simulink model "MDCC"  (R2021b)
settings: Solver=FixedStepDiscrete  StartTime=0.0  StopTime=10.0  FixedStep=0.0001  RelTol=1e-3
model workspace (MATLAB code in the model file):
  | cmdLim = Simulink.Parameter;
  | cmdLim.Value = 15;
  | cmdLim.Description = 'Limit for controlling the maximum surface command angle.';
  | cmdLim.Min = 0;
  | cmdLim.Max = 90;
  | cmdLim.DocUnits = 'deg';
  | 
  | dispGain = Simulink.Parameter;
  | dispGain.Value = 0.75;
  | dispGain.Description = 'Gain applied to the displacement error.';
  | dispGain.Min = 0;
  | dispGain.Max = [];
  | dispGain.DocUnits = 'deg/sec/deg';
  | 
  | dispLim = Simulink.Parameter;
  | dispLim.Value = 30;
  | dispLim.Description = 'Limit for controlling the maximum commanded angle.';
  | dispLim.Min = 0;
  | dispLim.Max = 180;
  | dispLim.DocUnits = 'deg';
  | 
  | intGain = Simulink.Parameter;
  | intGain.Value = 0.5;
  | intGain.Description = 'Gain applied to the integral error.';
  | intGain.Min = 0;
  | intGain.Max = [];
  | intGain.DocUnits = 'deg/sec/deg/sec';
  | 
  | intLim = Simulink.Parameter;
  | intLim.Value = 5;
  | intLim.Description = 'Limit for controlling the maximum commanded angle.';
  | intLim.Min = 0;
  | intLim.Max = 90;
  | intLim.DocUnits = 'deg';
  | 
  | rateGain = Simulink.Parameter;
  | rateGain.Value = 2;
  | rateGain.Description = 'Gain applied to the rate error.';
  | rateGain.Min = 0;
  | rateGain.Max = [];
  | rateGain.DocUnits = 'deg/deg/sec';
  | 
  | rateLim = Simulink.Parameter;
  | rateLim.Value = 6;
  | rateLim.Description = 'Limit for controlling the maximum commanded angle.';
  | rateLim.Min = 0;
  | rateLim.Max = 180;
  | rateLim.DocUnits = 'deg/sec';
  | 
  | hdgGain = Simulink.Parameter;
  | hdgGain.Value = 0.015;
values from neighbouring files (symbols this model uses):
  KfDeadCompen_SetDeltaTime_us = myPackage.Parameter    [DeadCompen.m]
  Ts = 5E-6    (= 5e-06)    [iPMSM_data.m]
  VbDeadComp_SwtUseIsttrDes_flg = myPackage.Parameter    [DeadCompen.m]
  VfDeadCompen_ISttrDdeThdSwt_A = myPackage.Parameter    [DeadCompen.m]
  VfDeadCompen_ISttrIgbtThdSwt_A = myPackage.Parameter    [DeadCompen.m]
  VfDeadCompen_rDdeISttrHi_R = myPackage.Parameter    [DeadCompen.m]
  VfDeadCompen_rDdeISttrLo_R = myPackage.Parameter    [DeadCompen.m]
  VfDeadCompen_rIgbtISttrHi_R = myPackage.Parameter    [DeadCompen.m]
  VfDeadCompen_rIgbtISttrLo_R = myPackage.Parameter    [DeadCompen.m]
  VfDeadCompen_uDdeISttrHi_V = myPackage.Parameter    [DeadCompen.m]
  VfDeadCompen_uDdeISttrLo_V = myPackage.Parameter    [DeadCompen.m]
  VfDeadCompen_uIgbtISttrHi_V = myPackage.Parameter    [DeadCompen.m]
  VfDeadCompen_uIgbtISttrLo_V = myPackage.Parameter    [DeadCompen.m]
undefined symbols (not defined in the file or in its folder): CosTable12bit_Y, GLBCal_GLBCal_Kf_DCLinkOverVolErrThd_V, GLBCal_GLBCal_Kf_DCLinkUnderVolErrThd_V, GLBCal_GLBCal_Kf_EquiLd_NULL, GLBCal_GLBCal_Kf_EquiLq_NULL, GLBCal_GLBCal_Kf_MotorRatedSpeed_rpm, GLBCal_GLBCal_Kf_MotorSpeedHysteresis_Coef, GLBCal_Ke_MotorPolePairsNum_NULL, IoHwAbOpArg_PwmDutyCyclePhU_NULL, IoHwAbOpArg_PwmDutyCyclePhV_NULL, IoHwAbOpArg_PwmDutyCyclePhW_NULL, IoHwAbOpArg_PwmOutputEn, KbMDCC_DeadTimeCompEn_flg, KbMDCC_MCF_flgHarmInIsdqTab11ZR_flg, KbMDCC_MCF_flgHarmInIsdqTab13ZR_flg, KbMDCC_MCF_flgHarmInIsdqTab5ZR_flg, KbMDCC_MCF_flgHarmInIsdqTab7ZR_flg, KbMDCC_MCF_flgHarmInject_flg, KbMDCC_SetEAngleEn_flg, KbMDCC_UdUqFwOmit_flg, KfDeadCompen_CpPeriodTimesT_NULL, KfMDCC_ActiveDischargeIdCurVal_A, KfMDCC_ActiveDischargeIqCurVal_A, KfMDCC_DCLinkVolRate_coef, KfMDCC_DebugEAngleInit_rad, KfMDCC_DebugUalphaVolCmd_V, KfMDCC_DebugUbetaVolCmd_V, KfMDCC_DebugUdCmd_V, KfMDCC_DebugUqCmd_V, KfMDCC_DebugUsCmd_V, KfMDCC_DebugUsRate_V, KfMDCC_IMCResp_NULL, KfMDCC_IMCStab_NULL, KfMDCC_InvParkCpPeriodTimesT_NULL, KfMDCC_MCF_CircAge_NULL, KfMDCC_MCF_flgUse11Harm_flg, KfMDCC_MCF_flgUse13Harm_flg, KfMDCC_MCF_flgUse5Harm_flg, KfMDCC_MCF_flgUse7Harm_flg, KfMDCC_MCF_Harm1113FLParamSpeedThrd_rads, KfMDCC_MCF_Harm57FLParamSpeedThrd_rads, KfMDCC_MCF_HarmcofFltN_NULL, KfMDCC_MCF_HarmCpnAg_NULL, KfMDCC_MCF_HarmfLParaHigh_coef, KfMDCC_MCF_HarmfLParaLow_coef, KfMDCC_MCF_HarmIn1113ZRY_Trq_Nm, KfMDCC_MCF_HarmIn11_SpdLimHigh_rads, KfMDCC_MCF_HarmIn11_SpdLimLow_rads, KfMDCC_MCF_HarmIn11ZRY_Isd_A, KfMDCC_MCF_HarmIn11ZRY_Isq_A, KfMDCC_MCF_HarmIn13_SpdLimHigh_rads, KfMDCC_MCF_HarmIn13_SpdLimLow_rads, KfMDCC_MCF_HarmIn13ZRY_Isd_A, KfMDCC_MCF_HarmIn13ZRY_Isq_A, KfMDCC_MCF_HarmIn57ZRY_Trq_Nm, KfMDCC_MCF_HarmIn5_SpdLimHigh_rads, KfMDCC_MCF_HarmIn5_SpdLimLow_rads, KfMDCC_MCF_HarmIn5ZRY_Isd_A, KfMDCC_MCF_HarmIn5ZRY_Isq_A, KfMDCC_MCF_HarmIn7_SpdLimHigh_rads ... (+47)
libraries: simulink x40, PMSM_Library x3, mcbcontrolslib x1
(part 1 of 8)
settings Model: RequirementInfo={} %GIDa_fe9045fd_0412_4b6e_8206_617cc20e6fde  DataDictionary=MDCC_Merge.sldd  FPTRunName=Active  Creator=洲  LastModifiedBy=洲
settings SolverCC: AlgebraicLoopSolver=TrustRegion  AutoInsertRateTranBlk=on
settings DataIOCC: SaveOutput=off  SignalLogging=off  DSMLogging=off  SaveTime=off
settings OptimizationCC: DefaultParameterBehavior=Inlined  UseDivisionForNetSlopeComputation=on  GainParamInheritBuiltInType=on  UseFloatMulNetSlope=on  DefaultUnderspecifiedDataType=single  UseSpecifiedMinMax=on  StrengthReduction=on  PassReuseOutputArgsAs=Individual arguments  ZeroExternalMemoryAtStartup=off  ZeroInternalMemoryAtStartup=off  NoFixptDivByZeroProtection=on  EfficientFloat2IntCast=on  OptimizeBlockOrder=speed  OptimizationPriority=Speed  OptimizationCustomize=off  MultiThreadedLoops=on  EfficientTunableParamExpr=on
settings DebuggingCC: ParameterTunabilityLossMsg=error  SFUnexpectedBacktrackingDiag=warning  SFNoUnconditionalDefaultTransitionDiag=warning  SFExecutionAtInitializationDiag=none  ArithmeticOperatorsInVariantConditions=warning
settings HardwareCC: ProdBitPerPointer=32  ProdBitPerSizeT=32  ProdBitPerPtrDiffT=32  ProdLargestAtomicInteger=Long  ProdLargestAtomicFloat=Double  ProdEndianess=BigEndian  ProdWordSize=32  ProdLongLongMode=on  ProdHWDeviceType=Freescale->32-bit PowerPC
settings ModelReferenceCC: ModelReferenceNumInstancesAllowed=Single
settings SFSimCC: MATLABDynamicMemAlloc=off  CustomCodeUndefinedFunction=UseInterfaceOnly
settings RTWCC: Description=AUTOSAR  SystemTargetFile=autosar.tlc  GenCodeOnly=on  TemplateMakefile=ert_default_tmf  BuildConfiguration=Faster Runs
settings CodeAppCC: ForceParamTrailComments=on  IgnoreCustomStorageClasses=off  MaxIdLength=128  OperatorAnnotations=on  SimulinkDataObjDesc=on  SFDataObjDesc=on  InsertBlockDesc=on  ReqsInCode=on
settings STFCustomTargetCC: TargetLangStandard=C99 (ISO)  UtilityFuncGeneration=Shared location  MultiwordLength=256  ParMdlRefBuildCompliant=on  CompOptLevelCompliant=on  IncludeMdlTerminateFcn=off  CombineOutputUpdateFcns=on  SuppressErrorStatus=on  ERTCustomFileBanners=on  SupportNonFinite=off  SupportComplex=off  SupportContinuousTime=off  SupportNonInlinedSFcns=off  RemoveResetFunc=on  MATLABClassNameForMDSCustomization=Simulink.SoftwareTarget.ERTCustomization  AutosarCompliant=on  GRTInterface=off  UseToolchainInfoCompliant=on  LookupTableObjectStructAxisOrder=2,1,3,4,...  LUTObjectStructOrderEvenSpacing=Size,Table,Breakpoints  SystemTargetFile=autosar.tlc
settings ERTTargetCC: TargetLangStandard=C99 (ISO)  UtilityFuncGeneration=Shared location  ConcurrentExecutionCompliant=off  IncludeMdlTerminateFcn=off  SuppressErrorStatus=on  SupportNonFinite=off  SupportComplex=off  ModelStepFunctionPrototypeControlCompliant=off  CPPClassGenCompliant=off  AutosarCompliant=on  LookupTableObjectStructAxisOrder=2,1,3,4,...  LUTObjectStructOrderEvenSpacing=Size,Table,Breakpoints  GenerateASAP2=on  InlinedParameterPlacement=NonHierarchical  ERTCustomFileTemplate=example_file_process.tlc
settings ConfigComp: CovScope=ReferencedModels  CovSaveName=covdata_rollAP  CovMetricSettings=dcmtrwe  CovHTMLOptions=-sRT=1 -aTS=1 -bRG=1 -bTC=1 -hTR=1 -nFC=0 -scm=1 -bcm=1 -xEv=0  CovSaveCumulativeToWorkspaceVar=on  CovSaveSingleToWorkspaceVar=on  CovCumulativeVarName=covCumulativeData_rollAP  CovReportOnPause=off  CovExternalEMLEnable=off  CovSFcnEnable=off

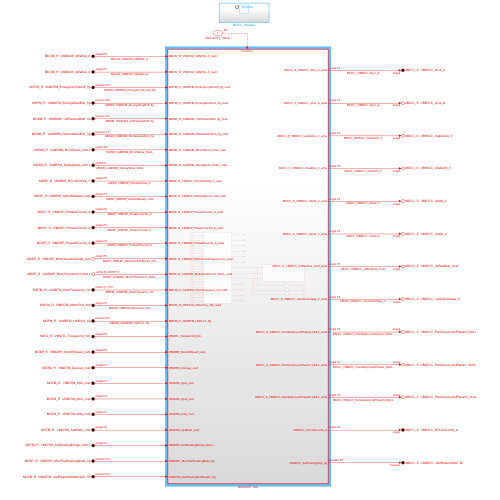
[thumbnail: Simulink's stored preview of the top-level diagram]
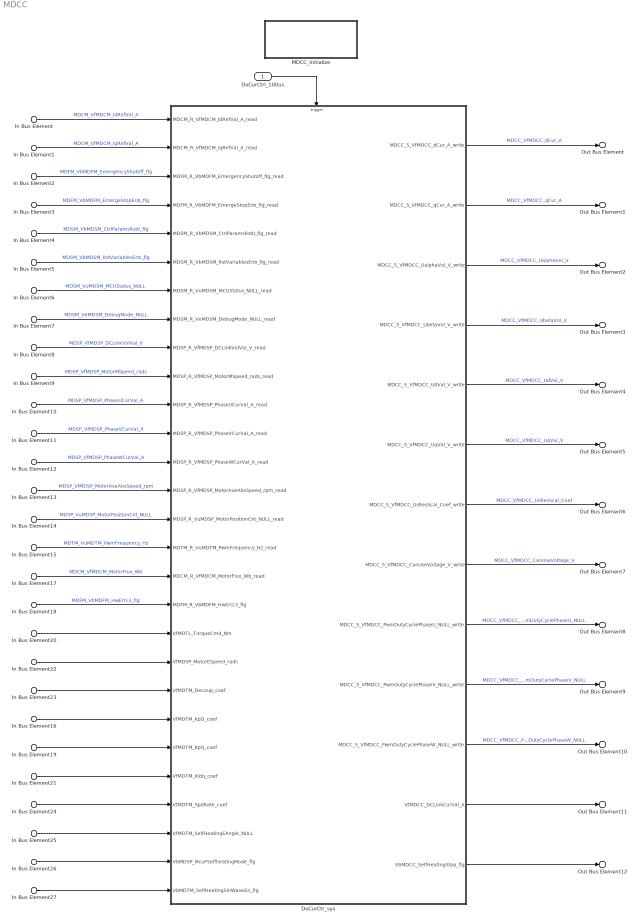
== system MDCC ==
  DoCurCtrl_100us : Inport  SampleTime=0.0001  OutputFunctionCall=on
  In Bus Element : Inport  Port=2  PortName=MDCM_R  Element=VfMDCM_IdRefVal_A
  In Bus Element1 : Inport  Port=2  PortName=MDCM_R  Element=VfMDCM_IqRefVal_A
  In Bus Element17 : Inport  Port=2  PortName=MDCM_R  Element=VfMDCM_MotorFlux_Wb
  In Bus Element2 : Inport  Port=3  PortName=MDFM_R  Element=VbMDFM_EmergencyShutoff_flg
  In Bus Element3 : Inport  Port=3  PortName=MDFM_R  Element=VbMDFM_EmergeStopEnb_flg
  In Bus Element18 : Inport  Port=3  PortName=MDFM_R  Element=VbMDFM_HwErrL3_flg
  In Bus Element4 : Inport  Port=4  PortName=MDSM_R  Element=VbMDSM_CtrlParamsRst0_flg
  In Bus Element5 : Inport  Port=4  PortName=MDSM_R  Element=VbMDSM_RstVariablesEnb_flg
  In Bus Element7 : Inport  Port=4  PortName=MDSM_R  Element=VeMDSM_DebugMode_NULL
  In Bus Element6 : Inport  Port=4  PortName=MDSM_R  Element=VuMDSM_MCUStatus_NULL
  In Bus Element26 : Inport  Port=5  PortName=MDSP_R  Element=VbMDSP_McuFSelfheatingMode_flg
  In Bus Element8 : Inport  Port=5  PortName=MDSP_R  Element=VfMDSP_DCLinkVolVal_V
  In Bus Element13 : Inport  Port=5  PortName=MDSP_R  Element=VfMDSP_MotorAveAbsSpeed_rpm
  In Bus Element22 : Inport  Port=5  PortName=MDSP_R  Element=VfMDSP_MotorESpeed_rads
  In Bus Element9 : Inport  Port=5  PortName=MDSP_R  Element=VfMDSP_MotorMSpeed_rads
  In Bus Element10 : Inport  Port=5  PortName=MDSP_R  Element=VfMDSP_PhaseUCurVal_A
  In Bus Element11 : Inport  Port=5  PortName=MDSP_R  Element=VfMDSP_PhaseVCurVal_A
  In Bus Element12 : Inport  Port=5  PortName=MDSP_R  Element=VfMDSP_PhaseWCurVal_A
  In Bus Element14 : Inport  Port=5  PortName=MDSP_R  Element=VuMDSP_MotorPositionCnt_NULL
  In Bus Element27 : Inport  Port=6  PortName=MDTM_R  Element=VbMDTM_SelfHeatingSinWaveEn_flg
  In Bus Element25 : Inport  Port=6  PortName=MDTM_R  Element=VfMDTM_SelfHeatingEAngle_NULL
  In Bus Element16 : Inport  Port=6  PortName=MDTM_R  Element=VfMDTM_KpD_coef
  In Bus Element19 : Inport  Port=6  PortName=MDTM_R  Element=VfMDTM_KpQ_coef
  In Bus Element21 : Inport  Port=6  PortName=MDTM_R  Element=VfMDTM_Kidq_coef
  In Bus Element23 : Inport  Port=6  PortName=MDTM_R  Element=VfMDTM_Decoup_coef
  In Bus Element24 : Inport  Port=6  PortName=MDTM_R  Element=VfMDTM_SpdRate_coef
  In Bus Element15 : Inport  Port=6  PortName=MDTM_R  Element=VuMDTM_PwmFrequency_Hz
  In Bus Element20 : Inport  Port=7  PortName=MDTL_R  Element=VfMDTL_TorqueCmd_Nm
  DoCurCtr_sys : Subsystem  Description=""
      settings: AttributesFormatString=%<Description>
  MDCC_Initialize : Subsystem  TreatAsAtomicUnit=on
  Out Bus Element12 : Outport  PortName=MDCC_S  Element=VbMDCC_SelfHeatingStop_flg
  Out Bus Element11 : Outport  PortName=MDCC_S  Element=VfMDCC_DCLinkCurVal_A
  Out Bus Element9 : Outport  PortName=MDCC_S  Element=VfMDCC_PwmDutyCyclePhaseV_NULL
  Out Bus Element7 : Outport  PortName=MDCC_S  Element=VfMDCC_CanUseVoltage_V
  Out Bus Element : Outport  PortName=MDCC_S  Element=VfMDCC_dCur_A
  Out Bus Element8 : Outport  PortName=MDCC_S  Element=VfMDCC_PwmDutyCyclePhaseU_NULL
  Out Bus Element10 : Outport  PortName=MDCC_S  Element=VfMDCC_PwmDutyCyclePhaseW_NULL
  Out Bus Element1 : Outport  PortName=MDCC_S  Element=VfMDCC_qCur_A
  Out Bus Element2 : Outport  PortName=MDCC_S  Element=VfMDCC_UalphaVol_V
  Out Bus Element3 : Outport  PortName=MDCC_S  Element=VfMDCC_UbetaVol_V
  Out Bus Element4 : Outport  PortName=MDCC_S  Element=VfMDCC_UdVal_V
  Out Bus Element5 : Outport  PortName=MDCC_S  Element=VfMDCC_UqVal_V
  Out Bus Element6 : Outport  PortName=MDCC_S  Element=VfMDCC_UsResScal_Coef
  wires:
  DoCurCtr_sys/10(MDCC_S_VfMDCC_PwmDutyCyclePhaseV_NULL_write) -> Out Bus Element9/1  "MDCC_VfMDCC_PwmDutyCyclePhaseV_NULL"
  DoCurCtr_sys/9(MDCC_S_VfMDCC_PwmDutyCyclePhaseU_NULL_write) -> Out Bus Element8/1  "MDCC_VfMDCC_PwmDutyCyclePhaseU_NULL"
  DoCurCtr_sys/3(MDCC_S_VfMDCC_UalphaVol_V_write) -> Out Bus Element2/1  "MDCC_VfMDCC_UalphaVol_V"
  In Bus Element14/1 -> DoCurCtr_sys/15(MDSP_R_VuMDSP_MotorPositionCnt_NULL_read)  "MDSP_VuMDSP_MotorPositionCnt_NULL"
  In Bus Element18/1 -> DoCurCtr_sys/18(MDFM_R_VbMDFM_HwErrL3_flg)  "MDFM_VbMDFM_HwErrL3_flg"
  DoCurCtr_sys/11(MDCC_S_VfMDCC_PwmDutyCyclePhaseW_NULL_write) -> Out Bus Element10/1  "MDCC_VfMDCC_PwmDutyCyclePhaseW_NULL"
  In Bus Element/1 -> DoCurCtr_sys/1(MDCM_R_VfMDCM_IdRefVal_A_read)  "MDCM_VfMDCM_IdRefVal_A"
  In Bus Element7/1 -> DoCurCtr_sys/8(MDSM_R_VeMDSM_DebugMode_NULL_read)  "MDSM_VeMDSM_DebugMode_NULL"
  In Bus Element11/1 -> DoCurCtr_sys/12(MDSP_R_VfMDSP_PhaseVCurVal_A_read)  "MDSP_VfMDSP_PhaseVCurVal_A"
  In Bus Element13/1 -> DoCurCtr_sys/14(MDSP_R_VfMDSP_MotorAveAbsSpeed_rpm_read)  "MDSP_VfMDSP_MotorAveAbsSpeed_rpm"
  DoCurCtr_sys/6(MDCC_S_VfMDCC_UqVal_V_write) -> Out Bus Element5/1  "MDCC_VfMDCC_UqVal_V"
  DoCurCtr_sys/4(MDCC_S_VfMDCC_UbetaVol_V_write) -> Out Bus Element3/1  "MDCC_VfMDCC_UbetaVol_V"
  In Bus Element1/1 -> DoCurCtr_sys/2(MDCM_R_VfMDCM_IqRefVal_A_read)  "MDCM_VfMDCM_IqRefVal_A"
  In Bus Element8/1 -> DoCurCtr_sys/9(MDSP_R_VfMDSP_DCLinkVolVal_V_read)  "MDSP_VfMDSP_DCLinkVolVal_V"
  DoCurCtr_sys/7(MDCC_S_VfMDCC_UsResScal_Coef_write) -> Out Bus Element6/1  "MDCC_VfMDCC_UsResScal_Coef"
  In Bus Element10/1 -> DoCurCtr_sys/11(MDSP_R_VfMDSP_PhaseUCurVal_A_read)  "MDSP_VfMDSP_PhaseUCurVal_A"
  DoCurCtr_sys/1(MDCC_S_VfMDCC_dCur_A_write) -> Out Bus Element/1  "MDCC_VfMDCC_dCur_A"
  In Bus Element9/1 -> DoCurCtr_sys/10(MDSP_R_VfMDSP_MotorMSpeed_rads_read)  "MDSP_VfMDSP_MotorMSpeed_rads"
  DoCurCtr_sys/5(MDCC_S_VfMDCC_UdVal_V_write) -> Out Bus Element4/1  "MDCC_VfMDCC_UdVal_V"
  In Bus Element12/1 -> DoCurCtr_sys/13(MDSP_R_VfMDSP_PhaseWCurVal_A_read)  "MDSP_VfMDSP_PhaseWCurVal_A"
  In Bus Element5/1 -> DoCurCtr_sys/6(MDSM_R_VbMDSM_RstVariablesEnb_flg_read)  "MDSM_VbMDSM_RstVariablesEnb_flg"
  In Bus Element17/1 -> DoCurCtr_sys/17(MDCM_R_VfMDCM_MotorFlux_Wb_read)  "MDCM_VfMDCM_MotorFlux_Wb"
  In Bus Element2/1 -> DoCurCtr_sys/3(MDFM_R_VbMDFM_EmergencyShutoff_flg_read)  "MDFM_VbMDFM_EmergencyShutoff_flg"
  DoCurCtr_sys/2(MDCC_S_VfMDCC_qCur_A_write) -> Out Bus Element1/1  "MDCC_VfMDCC_qCur_A"
  In Bus Element6/1 -> DoCurCtr_sys/7(MDSM_R_VuMDSM_MCUStatus_NULL_read)  "MDSM_VuMDSM_MCUStatus_NULL"
  In Bus Element4/1 -> DoCurCtr_sys/5(MDSM_R_VbMDSM_CtrlParamsRst0_flg_read)  "MDSM_VbMDSM_CtrlParamsRst0_flg"
  In Bus Element3/1 -> DoCurCtr_sys/4(MDFM_R_VbMDFM_EmergeStopEnb_flg_read)  "MDFM_VbMDFM_EmergeStopEnb_flg"
  DoCurCtr_sys/8(MDCC_S_VfMDCC_CanUseVoltage_V_write) -> Out Bus Element7/1  "MDCC_VfMDCC_CanUseVoltage_V"
  DoCurCtrl_100us/1 -> DoCurCtr_sys/Trigger
  In Bus Element15/1 -> DoCurCtr_sys/16(MDTM_R_VuMDTM_PwmFrequency_Hz_read)  "MDTM_VuMDTM_PwmFrequency_Hz"
  In Bus Element20/1 -> DoCurCtr_sys/19(VfMDTL_TorqueCmd_Nm)
  In Bus Element22/1 -> DoCurCtr_sys/20(VfMDSP_MotorESpeed_rads)
  DoCurCtr_sys/12(VfMDCC_DCLinkCurVal_A) -> Out Bus Element11/1
  In Bus Element23/1 -> DoCurCtr_sys/21(VfMDTM_Decoup_coef)
  In Bus Element16/1 -> DoCurCtr_sys/22(VfMDTM_KpD_coef)
  In Bus Element19/1 -> DoCurCtr_sys/23(VfMDTM_KpQ_coef)
  In Bus Element21/1 -> DoCurCtr_sys/24(VfMDTM_Kidq_coef)
  In Bus Element24/1 -> DoCurCtr_sys/25(VfMDTM_SpdRate_coef)
  In Bus Element25/1 -> DoCurCtr_sys/26(VfMDTM_SelfHeatingEAngle_NULL)
  In Bus Element26/1 -> DoCurCtr_sys/27(VbMDSP_McuFSelfheatingMode_flg)
  In Bus Element27/1 -> DoCurCtr_sys/28(VbMDTM_SelfHeatingSinWaveEn_flg)
  DoCurCtr_sys/13(VbMDCC_SelfHeatingStop_flg) -> Out Bus Element12/1

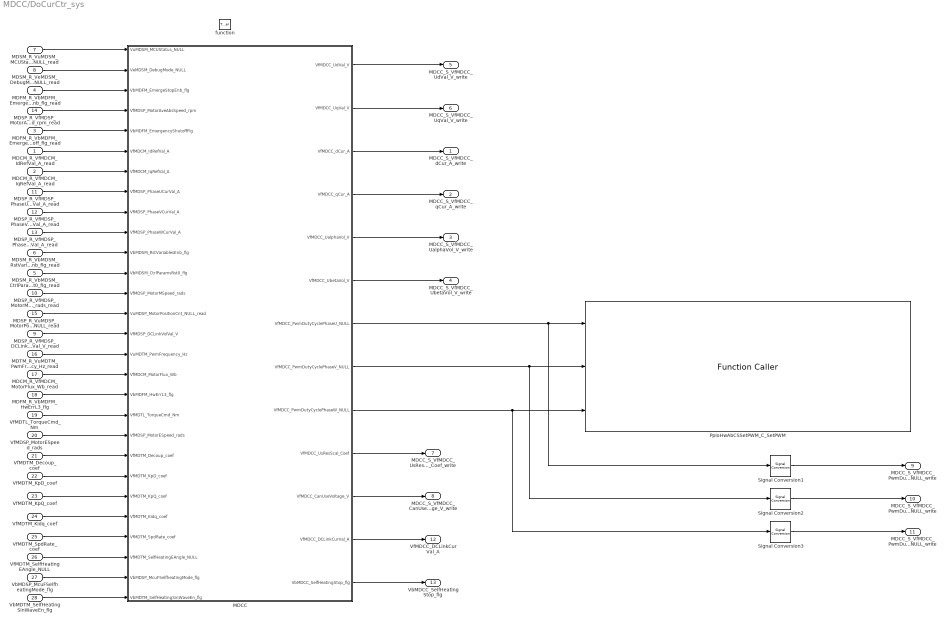
== system MDCC/DoCurCtr_sys ==
  MDCM_R_VfMDCM_IdRefVal_A_read : Inport
  MDCM_R_VfMDCM_IqRefVal_A_read : Inport  Port=2
  MDFM_R_VbMDFM_EmergencyShutoff_flg_read : Inport  Port=3
  MDFM_R_VbMDFM_EmergeStopEnb_flg_read : Inport  Port=4
  MDSM_R_VbMDSM_CtrlParamsRst0_flg_read : Inport  Port=5
  MDSM_R_VbMDSM_RstVariablesEnb_flg_read : Inport  Port=6
  MDSM_R_VuMDSM_MCUStatus_NULL_read : Inport  Port=7
  MDSM_R_VeMDSM_DebugMode_NULL_read : Inport  Port=8
  MDSP_R_VfMDSP_DCLinkVolVal_V_read : Inport  Port=9
  MDSP_R_VfMDSP_MotorMSpeed_rads_read : Inport  Port=10
  MDSP_R_VfMDSP_PhaseUCurVal_A_read : Inport  Port=11
  MDSP_R_VfMDSP_PhaseVCurVal_A_read : Inport  Port=12
  MDSP_R_VfMDSP_PhaseWCurVal_A_read : Inport  Port=13
  MDSP_R_VfMDSP_MotorAveAbsSpeed_rpm_read : Inport  Port=14
  MDSP_R_VuMDSP_MotorPositionCnt_NULL_read : Inport  Port=15
  MDTM_R_VuMDTM_PwmFrequency_Hz_read : Inport  Port=16  OutMin=1
  MDCM_R_VfMDCM_MotorFlux_Wb_read : Inport  Port=17
  MDFM_R_VbMDFM_HwErrL3_flg : Inport  Port=18
  VfMDTL_TorqueCmd_Nm : Inport  Port=19
  VfMDSP_MotorESpeed_rads : Inport  Port=20
  VfMDTM_Decoup_coef : Inport  Port=21
  VfMDTM_KpD_coef : Inport  Port=22
  VfMDTM_KpQ_coef : Inport  Port=23
  VfMDTM_Kidq_coef : Inport  Port=24
  VfMDTM_SpdRate_coef : Inport  Port=25
  VfMDTM_SelfHeatingEAngle_NULL : Inport  Port=26
  VbMDSP_McuFSelfheatingMode_flg : Inport  Port=27
  VbMDTM_SelfHeatingSinWaveEn_flg : Inport  Port=28
  function : TriggerPort  TriggerType=function-call  VariantControl=Variant  SampleTimeType=periodic  SampleTime=-1
  MDCC : Subsystem  RTWFcnName=MDCC  RTWFileName=MDCC
      settings: RTWSystemCode=Nonreusable function  RTWFcnNameOpts=User specified  RTWFileNameOpts=User specified  RTWMemSecFuncExecute=icache
  PpIoHwAbCSSetPWM_C_SetPWM : FunctionCaller  FunctionPrototype=PiIoHwSetPwmDuty_C_SwsSet_DPO_UVW_Duty(IoHwAbOpArg_PwmDutyCyclePhU_NULL,IoHwAbOpArg_PwmDutyCyclePhV_NULL,IoHwAbOpArg_PwmDutyCyclePhW_NULL)  InputArgumentSpecifications=single(0),single(0),single(0)
  Signal Conversion1 : SignalConversion  OverrideOpt=off
  Signal Conversion2 : SignalConversion  OverrideOpt=off
  Signal Conversion3 : SignalConversion  OverrideOpt=off
  MDCC_S_VfMDCC_dCur_A_write : Outport
  MDCC_S_VfMDCC_qCur_A_write : Outport  Port=2
  MDCC_S_VfMDCC_UalphaVol_V_write : Outport  Port=3
  MDCC_S_VfMDCC_UbetaVol_V_write : Outport  Port=4
  MDCC_S_VfMDCC_UdVal_V_write : Outport  Port=5
  MDCC_S_VfMDCC_UqVal_V_write : Outport  Port=6
  MDCC_S_VfMDCC_UsResScal_Coef_write : Outport  Port=7
  MDCC_S_VfMDCC_CanUseVoltage_V_write : Outport  Port=8
  MDCC_S_VfMDCC_PwmDutyCyclePhaseU_NULL_write : Outport  Port=9
  MDCC_S_VfMDCC_PwmDutyCyclePhaseV_NULL_write : Outport  Port=10
  MDCC_S_VfMDCC_PwmDutyCyclePhaseW_NULL_write : Outport  Port=11
  VfMDCC_DCLinkCurVal_A : Outport  Port=12
  VbMDCC_SelfHeatingStop_flg : Outport  Port=13
  wires:
  MDFM_R_VbMDFM_EmergencyShutoff_flg_read/1 -> MDCC/5(VbMDFM_EmergencyShutoffFlg)
  MDSM_R_VbMDSM_CtrlParamsRst0_flg_read/1 -> MDCC/12(VbMDSM_CtrlParamsRst0_flg)
  MDSM_R_VbMDSM_RstVariablesEnb_flg_read/1 -> MDCC/11(VbMDSM_RstVariablesEnb_flg)
  MDSP_R_VfMDSP_MotorMSpeed_rads_read/1 -> MDCC/13(VfMDSP_MotorMSpeed_rads)
  MDSP_R_VfMDSP_PhaseUCurVal_A_read/1 -> MDCC/8(VfMDSP_PhaseUCurVal_A)
  MDSP_R_VfMDSP_PhaseVCurVal_A_read/1 -> MDCC/9(VfMDSP_PhaseVCurVal_A)
  MDSP_R_VfMDSP_PhaseWCurVal_A_read/1 -> MDCC/10(VfMDSP_PhaseWCurVal_A)
  MDSP_R_VfMDSP_MotorAveAbsSpeed_rpm_read/1 -> MDCC/4(VfMDSP_MotorAveAbsSpeed_rpm)
  MDSP_R_VuMDSP_MotorPositionCnt_NULL_read/1 -> MDCC/14(VuMDSP_MotorPositionCnt_NULL_read)
  MDTM_R_VuMDTM_PwmFrequency_Hz_read/1 -> MDCC/16(VuMDTM_PwmFrequency_Hz)
  MDCC/7(VfMDCC_PwmDutyCyclePhaseU_NULL) -> Signal Conversion1/1, PpIoHwAbCSSetPWM_C_SetPWM/1
  MDCC/3(VfMDCC_dCur_A) -> MDCC_S_VfMDCC_dCur_A_write/1
  MDCC/4(VfMDCC_qCur_A) -> MDCC_S_VfMDCC_qCur_A_write/1
  MDCC/5(VfMDCC_UalphaVol_V) -> MDCC_S_VfMDCC_UalphaVol_V_write/1
  MDCC/6(VfMDCC_UbetaVol_V) -> MDCC_S_VfMDCC_UbetaVol_V_write/1
  MDCC/1(VfMDCC_UdVal_V) -> MDCC_S_VfMDCC_UdVal_V_write/1
  MDCC/2(VfMDCC_UqVal_V) -> MDCC_S_VfMDCC_UqVal_V_write/1
  MDCC/10(VfMDCC_UsResScal_Coef) -> MDCC_S_VfMDCC_UsResScal_Coef_write/1
  MDCC/11(VfMDCC_CanUseVoltage_V) -> MDCC_S_VfMDCC_CanUseVoltage_V_write/1
  MDCM_R_VfMDCM_MotorFlux_Wb_read/1 -> MDCC/17(VfMDCM_MotorFlux_Wb)
  MDFM_R_VbMDFM_EmergeStopEnb_flg_read/1 -> MDCC/3(VbMDFM_EmergeStopEnb_flg)
  MDSM_R_VuMDSM_MCUStatus_NULL_read/1 -> MDCC/1(VuMDSM_MCUStatus_NULL)
  MDSM_R_VeMDSM_DebugMode_NULL_read/1 -> MDCC/2(VeMDSM_DebugMode_NULL)
  Signal Conversion1/1 -> MDCC_S_VfMDCC_PwmDutyCyclePhaseU_NULL_write/1
  MDCC/8(VfMDCC_PwmDutyCyclePhaseV_NULL) -> Signal Conversion2/1, PpIoHwAbCSSetPWM_C_SetPWM/2
  Signal Conversion2/1 -> MDCC_S_VfMDCC_PwmDutyCyclePhaseV_NULL_write/1
  MDCC/9(VfMDCC_PwmDutyCyclePhaseW_NULL) -> Signal Conversion3/1, PpIoHwAbCSSetPWM_C_SetPWM/3
  Signal Conversion3/1 -> MDCC_S_VfMDCC_PwmDutyCyclePhaseW_NULL_write/1
  MDSP_R_VfMDSP_DCLinkVolVal_V_read/1 -> MDCC/15(VfMDSP_DCLinkVolVal_V)
  MDCM_R_VfMDCM_IdRefVal_A_read/1 -> MDCC/6(VfMDCM_IdRefVal_A)
  MDCM_R_VfMDCM_IqRefVal_A_read/1 -> MDCC/7(VfMDCM_IqRefVal_A)
  MDFM_R_VbMDFM_HwErrL3_flg/1 -> MDCC/18(VbMDFM_HwErrL3_flg)
  VfMDTL_TorqueCmd_Nm/1 -> MDCC/19(VfMDTL_TorqueCmd_Nm)
  VfMDSP_MotorESpeed_rads/1 -> MDCC/20(VfMDSP_MotorESpeed_rads)
  MDCC/12(VfMDCC_DCLinkCurVal_A) -> VfMDCC_DCLinkCurVal_A/1
  VfMDTM_Decoup_coef/1 -> MDCC/21(VfMDTM_Decoup_coef)
  VfMDTM_KpD_coef/1 -> MDCC/22(VfMDTM_KpD_coef)
  VfMDTM_KpQ_coef/1 -> MDCC/23(VfMDTM_KpQ_coef)
  VfMDTM_Kidq_coef/1 -> MDCC/24(VfMDTM_Kidq_coef)
  VfMDTM_SpdRate_coef/1 -> MDCC/25(VfMDTM_SpdRate_coef)
  VfMDTM_SelfHeatingEAngle_NULL/1 -> MDCC/26(VfMDTM_SelfHeatingEAngle_NULL)
  VbMDSP_McuFSelfheatingMode_flg/1 -> MDCC/27(VbMDSP_McuFSelfheatingMode_flg)
  VbMDTM_SelfHeatingSinWaveEn_flg/1 -> MDCC/28(VbMDTM_SelfHeatingSinWaveEn_flg)
  MDCC/13(VbMDCC_SelfHeatingStop_flg) -> VbMDCC_SelfHeatingStop_flg/1

== system MDCC/MDCC_Initialize ==
  Event Listener : EventListener  DisableCoverage=on  EventName=reset

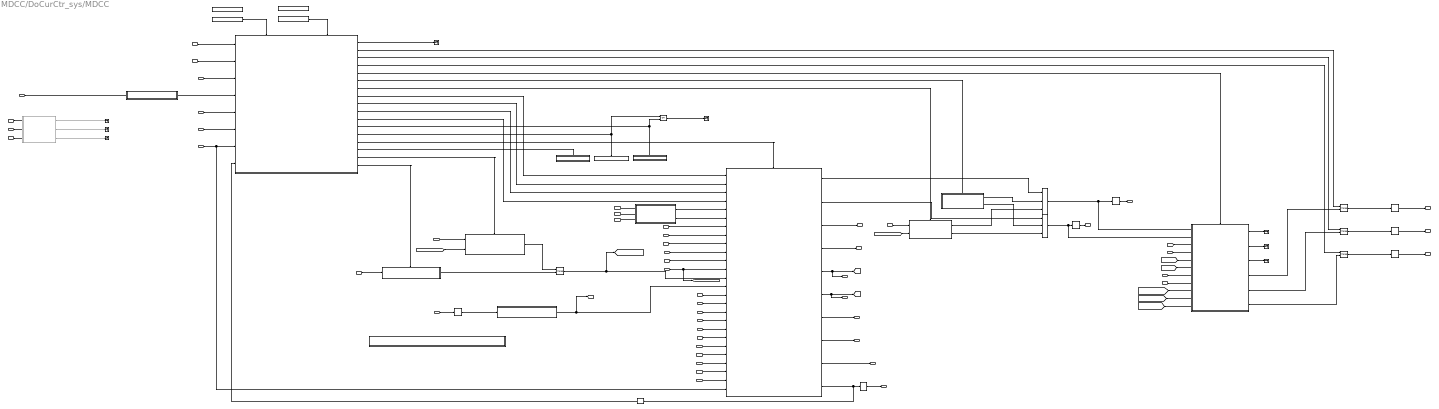
== system MDCC/DoCurCtr_sys/MDCC ==
  VuMDSM_MCUStatus_NULL : Inport
  VeMDSM_DebugMode_NULL : Inport  Port=2
  VbMDFM_EmergeStopEnb_flg : Inport  Port=3
  VfMDSP_MotorAveAbsSpeed_rpm : Inport  Port=4
  VbMDFM_EmergencyShutoffFlg : Inport  Port=5
  VfMDCM_IdRefVal_A : Inport  Port=6
  VfMDCM_IqRefVal_A : Inport  Port=7
  VfMDSP_PhaseUCurVal_A : Inport  Port=8
  VfMDSP_PhaseVCurVal_A : Inport  Port=9
  VfMDSP_PhaseWCurVal_A : Inport  Port=10
  VbMDSM_RstVariablesEnb_flg : Inport  Port=11
  VbMDSM_CtrlParamsRst0_flg : Inport  Port=12
  VfMDSP_MotorMSpeed_rads : Inport  Port=13
  VuMDSP_MotorPositionCnt_NULL_read : Inport  Port=14  OutMin=[0]  OutMax=[4095]
  VfMDSP_DCLinkVolVal_V : Inport  Port=15
  VuMDTM_PwmFrequency_Hz : Inport  Port=16
  VfMDCM_MotorFlux_Wb : Inport  Port=17
  VbMDFM_HwErrL3_flg : Inport  Port=18
  VfMDTL_TorqueCmd_Nm : Inport  Port=19
  VfMDSP_MotorESpeed_rads : Inport  Port=20
  VfMDTM_Decoup_coef : Inport  Port=21
  VfMDTM_KpD_coef : Inport  Port=22
  VfMDTM_KpQ_coef : Inport  Port=23
  VfMDTM_Kidq_coef : Inport  Port=24
  VfMDTM_SpdRate_coef : Inport  Port=25
  VfMDTM_SelfHeatingEAngle_NULL : Inport  Port=26
  VbMDSP_McuFSelfheatingMode_flg : Inport  Port=27
  VbMDTM_SelfHeatingSinWaveEn_flg : Inport  Port=28
  AND : Logic  Operator=OR  AllPortsSameDT=off  OutDataTypeStr=boolean
  ASC : Subsystem  TreatAsAtomicUnit=on
  ASCSpeedHysteresis_Sys : Subsystem
  ActiveDischarge_Sys : Subsystem
  DCLinkLimit_Sys : Subsystem  TreatAsAtomicUnit=on
      settings: RTWSystemCode=Nonreusable function  RTWFcnNameOpts=Use subsystem name
  Data Store Memory : DataStoreMemory  DataStoreName=MDSP_VbMDSP_HardwareASC_flg  ReadBeforeWriteMsg=warning  WriteAfterWriteMsg=warning  WriteAfterReadMsg=warning  ShowAdditionalParam=off  StateMustResolveToSignalObject=on
  Data Store Memory1 : DataStoreMemory  DataStoreName=MDSP_VbMDSP_HardwareFW_flg  ReadBeforeWriteMsg=warning  WriteAfterWriteMsg=warning  WriteAfterReadMsg=warning  ShowAdditionalParam=off  StateMustResolveToSignalObject=on
  Data Store Read : DataStoreRead  DataStoreName=MDSP_VbMDSP_HardwareFW_flg  IndexOptions=Index vector (dialog)  Indices=1  OutputSizes=1
  Data Store Read1 : DataStoreRead  DataStoreName=MDSP_VbMDSP_HardwareASC_flg  IndexOptions=Index vector (dialog)  Indices=1  OutputSizes=1
  Delay : Delay  DelayLength=1
  EAngleSetFixVal_Sys : Subsystem
      settings: RTWSystemCode=Nonreusable function  RTWFcnNameOpts=Use subsystem name
  FW : Subsystem  TreatAsAtomicUnit=on
  IrmsCalc_Sys : Subsystem  Commented=on  TreatAsAtomicUnit=on  RTWFcnName=IrmsCalc
      settings: RTWSystemCode=Nonreusable function  RTWFcnNameOpts=User specified
  MDCC_Debug_UaUb : Subsystem  TreatAsAtomicUnit=on
      settings: RTWSystemCode=Nonreusable function  RTWFcnNameOpts=Use subsystem name
  MDCC_Debug_Us : Subsystem  TreatAsAtomicUnit=on
      settings: RTWSystemCode=Nonreusable function  RTWFcnNameOpts=Use subsystem name
  MDCC_State : Stateflow chart  TreatAsAtomicUnit=on
      settings: RTWSystemCode=Nonreusable function  RTWFcnNameOpts=Use subsystem name  PortSchema="{\"entries\":[{\"content\":{\"sides\":[{\"content\":{\"connectorIds\":[\"In3\",\"In4\",\"In5\",\"In6\",\"In7\",\"In8\",\"In9\",\"In10\"]},\"type\":\"ConnectorPlacement.EquallySpacedRectSide\",\"uuid\":\"6c31981e-4ed7-4699-b2ce-c12c69aaec8a\"},{\"content\":{\"connectorIds\":[\"Out1\",\"Out2\",\"Out3\",\"Out4\",\"Out11\",\"Out12\",\"Out13\",\"Out5\",\"Out6\",\"Out10\",\"Out7\",\"Out9\",\"Out8\",\"Out14\",\"Out15\",\"Out16\",\"Out17\"],\"side\":\"RIGHT\"},\"type\":\"ConnectorPlacement.EquallySpacedRectSide\",\"uuid\":\"a74e42ce-bc1d-4148-a54f-622647aedd35\"},{\"content\":{\"connectorIds\":[\"In1\",\"In2\"],\"side\":\"TOP\"},\"type\":\"ConnectorPlacement.EquallySpacedRectSide\",\"uuid\":\"88987904-7cee-4481-9b83-2a51868102e1\"}]},\"type\":\"ConnectorPlacement.EquallySpacedConnector\",\"uuid\":\"06e2d35e-b9db-42d1-b1d9-c7ee8e17a460\"}],\"packageUris\":[\"http://schema.mathworks.com/mf0/Connector/R2020b\"],\"version\":\"1.0\"}"
  Merge : Merge  Inputs=3
  Merge1 : Merge  Inputs=3
  Merge{2..5} (4 alike) : Merge
  PWMEn : Subsystem
  ResAngle_Sys : Subsystem
  SVM_Calc : Subsystem
      settings: RTWSystemCode=Nonreusable function  RTWFcnNameOpts=Use subsystem name
  Signal Conversion{2..6} (5 alike) : SignalConversion  OverrideOpt=off
  Signal Copy : SignalConversion  OverrideOpt=off
  Signal Copy1 : SignalConversion  OverrideOpt=off
  Simulink Function : Subsystem  TreatAsAtomicUnit=on
  Terminator{,1..7} (8 alike) : Terminator
  UdUqCalc_Sys : Subsystem  TreatAsAtomicUnit=on  RTWFcnName=vPwm_MDCC_UdUqCalc1  RTWFileName=MDCC
      settings: RTWSystemCode=Nonreusable function  RTWFcnNameOpts=User specified
  VfMDCM_IdRefVal_A1 : InportShadow  Port=6
  VfMDCM_IqRefVal_A1 : InportShadow  Port=7
  VfMDSP_PhaseUCurVal_A1 : InportShadow  Port=8
  VfMDSP_PhaseVCurVal_A1 : InportShadow  Port=9
  VfMDSP_PhaseWCurVal_A1 : InportShadow  Port=10
  VuMDSM_MCUStatus_NULL1 : InportShadow
  VuMDTM_PwmFrequency_Hz1 : InportShadow  Port=16
  VuMDTM_PwmFrequency_Hz2 : InportShadow  Port=16
  VuMDTM_PwmFrequency_Hz3 : InportShadow  Port=16
  VfMDCC_UdVal_V : Outport
  VfMDCC_UqVal_V : Outport  Port=2
  VfMDCC_dCur_A : Outport  Port=3
  VfMDCC_qCur_A : Outport  Port=4
  VfMDCC_UalphaVol_V : Outport  Port=5
  VfMDCC_UbetaVol_V : Outport  Port=6
  VfMDCC_PwmDutyCyclePhaseU_NULL : Outport  Port=7
  VfMDCC_PwmDutyCyclePhaseV_NULL : Outport  Port=8
  VfMDCC_PwmDutyCyclePhaseW_NULL : Outport  Port=9
  VfMDCC_UsResScal_Coef : Outport  Port=10
  VfMDCC_CanUseVoltage_V : Outport  Port=11
  VfMDCC_DCLinkCurVal_A : Outport  Port=12
  VbMDCC_SelfHeatingStop_flg : Outport  Port=13
  wires:
  Merge/1 -> SVM_Calc/1(VfMDCC_UalphaVol_V), Signal Conversion2/1  "VfMDCC_UalphaVol_V"
  Merge1/1 -> Signal Conversion3/1, SVM_Calc/2(VfMDCC_UbetaVol_V)  "VfMDCC_UbetaVol_V"
  UdUqCalc_Sys/1(VfMDCC_UalphaVol_V) -> Merge/1
  UdUqCalc_Sys/3(VfMDCC_UdVal_V) -> VfMDCC_UdVal_V/1
  UdUqCalc_Sys/4(VfMDCC_UqVal_V) -> VfMDCC_UqVal_V/1
  Merge2/1 -> Signal Conversion4/1  "VfMDCC_PwmDutyCyclePhaseU_NULL"
  Merge4/1 -> Signal Conversion6/1  "VfMDCC_PwmDutyCyclePhaseW_NULL"
  Merge3/1 -> Signal Conversion5/1  "VfMDCC_PwmDutyCyclePhaseV_NULL"
  MDCC_State/1(VeMDSM_PWMOutMode_enum) -> Terminator4/1  "VeMDSM_PWMOutMode_enum"
  MDCC_State/14(UdUqCalc()) -> UdUqCalc_Sys/Trigger
  MDCC_State/5(VbMDCC_UdUqCalc1Enb_flg) -> UdUqCalc_Sys/1(VbMDCC_UdUqCalc1Enb_flg)
  MDCC_State/6(VbMDCC_UdUqCalc2Enb_flg) -> UdUqCalc_Sys/2(VbMDCC_UdUqCalc2Enb_flg)
  VbMDSM_RstVariablesEnb_flg/1 -> UdUqCalc_Sys/10(VbMDSM_RstVariablesEnb_flg)
  VbMDSM_CtrlParamsRst0_flg/1 -> UdUqCalc_Sys/11(VbMDSM_CtrlParamsRst0_flg)
  MDCC_State/12(MDCC_DebugUaUb_Call()) -> MDCC_Debug_UaUb/Trigger
  MDCC_Debug_UaUb/1(VfMDCC_UalphaVol_V) -> Merge/2
  MDCC_Debug_UaUb/2(VfMDCC_UbetaVol_V) -> Merge1/2
  VfMDSP_PhaseUCurVal_A/1 -> UdUqCalc_Sys/7(VfMDSP_PhaseUCurVal_A)
  VfMDSP_PhaseVCurVal_A/1 -> UdUqCalc_Sys/8(VfMDSP_PhaseVCurVal_A)
  VfMDSP_PhaseWCurVal_A/1 -> UdUqCalc_Sys/9(VfMDSP_PhaseWCurVal_A)
  MDCC_State/2(VfMDSA_PwmDutyCyclePhaseU_NULL) -> Merge2/1
  MDCC_State/3(VfMDSA_PwmDutyCyclePhaseV_NULL) -> Merge3/1
  MDCC_State/4(VfMDSA_PwmDutyCyclePhaseW_NULL) -> Merge4/1
  VuMDTM_PwmFrequency_Hz/1 -> UdUqCalc_Sys/15(ui16_Pwm_Freq)
  VbMDFM_EmergeStopEnb_flg/1 -> MDCC_State/5(VbMDFM_EmergeStopEnb_flg)
  VbMDFM_EmergencyShutoffFlg/1 -> MDCC_State/7(VbMDFM_EmergencyShutoff_flg)
  MDCC_State/13(MDCC_DebugUs_Call()) -> MDCC_Debug_Us/Trigger
  VuMDTM_PwmFrequency_Hz1/1 -> MDCC_Debug_Us/1(VuMDTM_PwmFrequency_Hz)
  MDCC_Debug_Us/2(VfMDCC_UbetaVol_V) -> Merge1/3
  MDCC_Debug_Us/1(VfMDCC_UalphaVol_V) -> Merge/3
  UdUqCalc_Sys/2(VfMDCC_UbetaVol_V) -> Merge1/1
  UdUqCalc_Sys/5(VfMDCC_dCur_A) -> VfMDCC_dCur_A/1, [VfMDCC_dCur_A]
  UdUqCalc_Sys/6(VfMDCC_qCur_A) -> VfMDCC_qCur_A/1, [VfMDCC_qCur_A]
  Signal Conversion2/1 -> VfMDCC_UalphaVol_V/1
  Signal Conversion3/1 -> VfMDCC_UbetaVol_V/1
  Signal Conversion4/1 -> VfMDCC_PwmDutyCyclePhaseU_NULL/1
  Signal Conversion5/1 -> VfMDCC_PwmDutyCyclePhaseV_NULL/1
  Signal Conversion6/1 -> VfMDCC_PwmDutyCyclePhaseW_NULL/1
  UdUqCalc_Sys/7(VfMDCC_UsResScal_Coef) -> VfMDCC_UsResScal_Coef/1
  UdUqCalc_Sys/8(VfMDCC_CanUseVoltage_V) -> VfMDCC_CanUseVoltage_V/1
  VfMDCM_MotorFlux_Wb/1 -> UdUqCalc_Sys/16(VfMDCM_MotorFlux_Wb)
  MDCC_State/11(MDCC_MDSA_Call()) -> SVM_Calc/Trigger
  SVM_Calc/4(VfMDCC_PWMDutyUDeadCompFINAL_NULL) -> Merge2/2
  SVM_Calc/5(VfMDCC_PWMDutyVDeadCompFINAL_NULL) -> Merge3/2
  SVM_Calc/6(VfMDCC_PWMDutyWDeadCompFINAL_NULL) -> Merge4/2
  MDCC_State/7(VbMDCC_PIRstEn_flg) -> UdUqCalc_Sys/4(VbMDCC_PIRstEn_flg)  "VbMDCC_PIRstEn_flg"
  MDCC_State/15(MDCC_FW_Call()) -> FW/Trigger
  Merge5/1 -> [VuMDCC_MotorPositionCnt_NULL], UdUqCalc_Sys/13(VuMDCC_MotorPositionCnt_NULL)  "VuMDCC_MotorPositionCnt_NULL"
  DCLinkLimit_Sys/1(VfMDCC_DCLinkVolUsed_V) -> UdUqCalc_Sys/14(VfMDCC_DCLinkVolUsed_V), [VfMDCC_DCLinkVolUsed_V_Tag]  "VfMDCC_DCLinkVolUsed_V"
  Signal Copy1/1 -> DCLinkLimit_Sys/1(VfMDSP_DCLinkVolVal_V)  "VfMDSP_DCLinkVolVal_V"
  MDCC_State/16(AutoEAngle_Calc()) -> EAngleSetFixVal_Sys/Trigger
  MDCC_State/17(ResEAngle_Calc()) -> ResAngle_Sys/Trigger
  EAngleSetFixVal_Sys/1(VuMDCC_MotorPositionCnt_NULL) -> Merge5/1
  ResAngle_Sys/1(VuMDCC_MotorPositionCnt_NULL) -> Merge5/2
  VfMDSP_MotorMSpeed_rads/1 -> [VfMDSP_MotorMSpeed_rads_Tag], UdUqCalc_Sys/12(VfMDSP_MotorMSpeed_rads)
  VuMDSP_MotorPositionCnt_NULL_read/1 -> ResAngle_Sys/1(VuMDSP_MotorPositionCnt_NULL_read)
  VuMDTM_PwmFrequency_Hz2/1 -> EAngleSetFixVal_Sys/1(VuMDTM_PwmFrequency_Hz)
  [VfMDCC_DCLinkVolUsed_V_Tag] -> SVM_Calc/3(VfMDCC_DCLinkVolUsed_V)
  VuMDTM_PwmFrequency_Hz3/1 -> SVM_Calc/4(VuMDTM_PwmFrequency_Hz)
  VbMDFM_HwErrL3_flg/1 -> MDCC_State/8(VbMDFM_HwErrL3_flg)
  VfMDCM_IdRefVal_A1/1 -> SVM_Calc/7(VfMDCM_IdRefVal_A)
  VfMDCM_IqRefVal_A1/1 -> SVM_Calc/8(VfMDCM_IqRefVal_A)
  [VfMDCC_qCur_A] -> SVM_Calc/6(VfMDCC_qCur_A)
  [VfMDCC_dCur_A] -> SVM_Calc/5(VfMDCC_dCur_A)
  SVM_Calc/1(VfMDCC_PwmDutyCyclePhaseU_NULL) -> Terminator/1
  SVM_Calc/2(VfMDCC_PwmDutyCyclePhaseV_NULL) -> Terminator1/1
  SVM_Calc/3(VfMDCC_PwmDutyCyclePhaseW_NULL) -> Terminator2/1
  VuMDSM_MCUStatus_NULL1/1 -> ActiveDischarge_Sys/1(VuMDSM_MCUStatus_NULL)
  VfMDCM_IdRefVal_A/1 -> ActiveDischarge_Sys/2(VfMDCM_IdRefVal_A)
  VfMDCM_IqRefVal_A/1 -> ActiveDischarge_Sys/3(VfMDCM_IqRefVal_A)
  ActiveDischarge_Sys/1(VfMDCC_IdRefVal_A) -> UdUqCalc_Sys/5(VfMDCC_IdRefVal_A)
  ActiveDischarge_Sys/2(VfMDCC_IqRefVal_A) -> UdUqCalc_Sys/6(VfMDCC_IqRefVal_A)
  VfMDSP_MotorESpeed_rads/1 -> UdUqCalc_Sys/18(VfMDSP_MotorESpeed_rads)
  VfMDTL_TorqueCmd_Nm/1 -> UdUqCalc_Sys/17(VfMDTL_TorqueCmd_Nm)
  VuMDSM_MCUStatus_NULL/1 -> MDCC_State/3(VuMDSM_MCUStatus_NULL)
  VeMDSM_DebugMode_NULL/1 -> MDCC_State/4(VeMDST_MDSMDebugMode_NULL)
  MDCC_State/9(VbMDCC_ASCEnable_flg) -> AND/2, ASC/Trigger
  VfMDSP_MotorAveAbsSpeed_rpm/1 -> ASCSpeedHysteresis_Sys/1(VfMDCC_MotorAveAbsSpeed_rpm)
  ASCSpeedHysteresis_Sys/1(VbMDCC_MotorASCEn_flg) -> MDCC_State/6(VbMDCC_MotorASCEn_flg)  "MDCC_VbMDCC_MotorASCEn_flg"
  UdUqCalc_Sys/9(VfMDCC_DCLinkCurVal_A) -> VfMDCC_DCLinkCurVal_A/1
  [VfMDSP_MotorMSpeed_rads_Tag] -> EAngleSetFixVal_Sys/2(VfMDSP_MotorMSpeed_rads)
  [VfMDSP_MotorMSpeed_rads_Tag] -> MDCC_Debug_Us/2(VfMDSP_MotorMSpeed_rads)
  VfMDTM_Decoup_coef/1 -> UdUqCalc_Sys/19(VfMDTM_Decoup_coef)
  VfMDTM_KpQ_coef/1 -> UdUqCalc_Sys/21(VfMDTM_KpQ_coef)
  VfMDTM_SpdRate_coef/1 -> UdUqCalc_Sys/23(VfMDTM_SpdRate_coef)
  VfMDTM_KpD_coef/1 -> UdUqCalc_Sys/20(VfMDTM_KpD_coef)
  VfMDTM_Kidq_coef/1 -> UdUqCalc_Sys/22(VfMDTM_Kidq_coef)
  VbMDSP_McuFSelfheatingMode_flg/1 -> MDCC_State/9(VbMDSP_McuFSelfheatingMode_flg), UdUqCalc_Sys/26(VbMDSP_McuFSelfheatingMode_flg)
  VfMDTM_SelfHeatingEAngle_NULL/1 -> UdUqCalc_Sys/24(VfMDTM_SelfHeatingEAngle_NULL)
  MDCC_State/10(VbMDCC_SelfHeatingEn_flg) -> UdUqCalc_Sys/3(VbMDCC_SelfHeatingEn_flg)
  VbMDTM_SelfHeatingSinWaveEn_flg/1 -> UdUqCalc_Sys/25(VbMDTM_SelfHeatingSinWaveEn_flg)
  UdUqCalc_Sys/10(VbMDCC_SelfHeatingStop_flg) -> Delay/1, Signal Copy/1  "MDCC_VbMDCC_SelfHeatingStop_flg"
  Delay/1 -> MDCC_State/10(VbMDCC_PreSelfHeatingStop_flg)
  MDCC_State/8(MDCC_PWMEn) -> AND/1, PWMEn/Trigger
  AND/1 -> Terminator7/1  "MDCC_VbMDCC_EopStartEn_flg"
  Data Store Read/1 -> MDCC_State/1(MDSP_VbMDSP_HardwareFW_flg)
  Data Store Read1/1 -> MDCC_State/2(MDSP_VbMDSP_HardwareASC_flg)
  VfMDSP_PhaseUCurVal_A1/1 -> IrmsCalc_Sys/1(A_Element_Inlet)
  VfMDSP_PhaseVCurVal_A1/1 -> IrmsCalc_Sys/2(B_Element_Inlet)
  VfMDSP_PhaseWCurVal_A1/1 -> IrmsCalc_Sys/3(C_Element_Inlet)
  IrmsCalc_Sys/1(A_Rms_Out) -> Terminator3/1  "MDCC_VfMDCC_PhaseUCurRmsVal_A"
  IrmsCalc_Sys/2(B_Rms_Out) -> Terminator5/1  "MDCC_VfMDCC_PhaseVCurRmsVal_A"
  IrmsCalc_Sys/3(C_Rms_Out) -> Terminator6/1  "MDCC_VfMDCC_PhaseWCurRmsVal_A"
  Signal Copy/1 -> VbMDCC_SelfHeatingStop_flg/1
  VfMDSP_DCLinkVolVal_V/1 -> Signal Copy1/1
  [VfMDSP_MotorMSpeed_rads_Tag] -> SVM_Calc/10(VfMDSP_MotorMSpeed_rads)
  [VfMDCC_DCLinkVolUsed_V_Tag] -> SVM_Calc/11(uDcLink)
  [VuMDCC_MotorPositionCnt_NULL] -> SVM_Calc/9(VuMDSP_MotorPositionCnt_NULL)

== system MDCC/DoCurCtr_sys/MDCC/ASC ==
  FCN : TriggerPort  VariantControl=(inherit)  PortDimensions=1
  CDD_Gtm_UVW_SetAsc : FunctionCaller  FunctionPrototype=PiIoHwSetInvState_C_SwsSet_DPO_UVW_Asc()  InputArgumentSpecifications=<Enter example>  OutputArgumentSpecifications=<Enter example>

== system MDCC/DoCurCtr_sys/MDCC/ASCSpeedHysteresis_Sys ==
  VfMDCC_MotorAveAbsSpeed_rpm : Inport
  Add1 : Sum  Inputs=+-
  Constant : Constant  Value=GLBCal_GLBCal_Kf_MotorRatedSpeed_rpm
  Constant6 : Constant  Value=boolean(0)
  Constant7 : Constant  Value=boolean(1)
  Constant8 : Constant  Value=GLBCal_GLBCal_Kf_MotorSpeedHysteresis_Coef  OutDataTypeStr=single
  LowPowerOverVolErrM_L2 : PMSM_Library/RelayModified  SystemSampleTime=-1  VariantActivationTime=update diagram  Latency=0  AutoFrameSizeCalculation=off
  VbMDCC_MotorASCEn_flg : Outport
  wires:
  Constant7/1 -> LowPowerOverVolErrM_L2/4
  LowPowerOverVolErrM_L2/1 -> VbMDCC_MotorASCEn_flg/1
  Constant6/1 -> LowPowerOverVolErrM_L2/5
  Constant8/1 -> Add1/2
  Add1/1 -> LowPowerOverVolErrM_L2/3
  Constant/1 -> LowPowerOverVolErrM_L2/2, Add1/1
  VfMDCC_MotorAveAbsSpeed_rpm/1 -> LowPowerOverVolErrM_L2/1

== system MDCC/DoCurCtr_sys/MDCC/ActiveDischarge_Sys ==
  VuMDSM_MCUStatus_NULL : Inport
  VfMDCM_IdRefVal_A : Inport  Port=2
  VfMDCM_IqRefVal_A : Inport  Port=3
  Constant : Constant  Value=KfMDCC_ActiveDischargeIdCurVal_A
  Constant1 : Constant  Value=KfMDCC_ActiveDischargeIqCurVal_A
  Data Type Conversion : DataTypeConversion  OutDataTypeStr=uint16
  Enumerated Constant2 : simulink/Sources/Enumerated Constant  OutDataTypeStr=Enum: MDSM_MCUStatus  Value=MDSM_MCUStatus.MDSM_ActiveDischarge  SampleTime=inf
  Relational Operator : RelationalOperator  Operator===  OutDataTypeStr=boolean  RndMeth=Simplest
  Switch : Switch  Criteria=u2 ~= 0
  Switch1 : Switch  Criteria=u2 ~= 0
  VfMDCC_IdRefVal_A : Outport
  VfMDCC_IqRefVal_A : Outport  Port=2
  wires:
  VfMDCM_IqRefVal_A/1 -> Switch1/3
  Relational Operator/1 -> Switch/2, Switch1/2
  Enumerated Constant2/1 -> Data Type Conversion/1
  VfMDCM_IdRefVal_A/1 -> Switch/3
  Switch1/1 -> VfMDCC_IqRefVal_A/1
  Switch/1 -> VfMDCC_IdRefVal_A/1
  VuMDSM_MCUStatus_NULL/1 -> Relational Operator/2
  Constant1/1 -> Switch1/1
  Constant/1 -> Switch/1
  Data Type Conversion/1 -> Relational Operator/1

== system MDCC/DoCurCtr_sys/MDCC/DCLinkLimit_Sys ==
  VfMDSP_DCLinkVolVal_V : Inport
  Constant2 : Constant  Value=GLBCal_GLBCal_Kf_DCLinkUnderVolErrThd_V
  Constant3 : Constant  Value=GLBCal_GLBCal_Kf_DCLinkOverVolErrThd_V
  Saturation Dynamic : simulink/Discontinuities/Saturation Dynamic  OutMin=[]  OutMax=[]  OutDataTypeStr=Inherit: Same as second input  OutDataType=fixdt(1, 16)  OutScaling=2^-10  DoSatur=off
  VfMDCC_DCLinkVolUsed_V : Outport
  wires:
  Constant3/1 -> Saturation Dynamic/1
  Constant2/1 -> Saturation Dynamic/3
  VfMDSP_DCLinkVolVal_V/1 -> Saturation Dynamic/2
  Saturation Dynamic/1 -> VfMDCC_DCLinkVolUsed_V/1

== system MDCC/DoCurCtr_sys/MDCC/EAngleSetFixVal_Sys ==
  VuMDTM_PwmFrequency_Hz : Inport
  VfMDSP_MotorMSpeed_rads : Inport  Port=2
  FCN : TriggerPort  TriggerType=function-call  VariantControl=(inherit)  PortDimensions=1
  Constant : Constant  Value=KbMDCC_SetEAngleEn_flg
  Constant4 : Constant  Value=KuMDCC_SetEAngle_Null  OutMin=0  OutMax=360  OutDataTypeStr=single
  GLBCal_Ke_MotorPolePairsNum_NULL : Constant  Value=GLBCal_Ke_MotorPolePairsNum_NULL
  Ku_EAngleSet_Caller : FunctionCaller  FunctionPrototype=Vu_AutoEAngle_NULL = Ku_EAngleSet(Kf_SpdCmd_rads,Vu_PwmFrequency_Hz,Ke_MotorPolePairsNum_NULL,Kb_SetEAngleFixValEn_flg,Kf_SetEAngle_Null)  InputArgumentSpecifications=single(0),uint16(0),uint8(0),boolean(0),single(0)  OutputArgumentSpecifications=uint16(0)
  VuMDCC_MotorPositionCnt_NULL : Outport
  wires:
  VuMDTM_PwmFrequency_Hz/1 -> Ku_EAngleSet_Caller/2
  GLBCal_Ke_MotorPolePairsNum_NULL/1 -> Ku_EAngleSet_Caller/3
  Ku_EAngleSet_Caller/1 -> VuMDCC_MotorPositionCnt_NULL/1
  Constant/1 -> Ku_EAngleSet_Caller/4
  Constant4/1 -> Ku_EAngleSet_Caller/5
  VfMDSP_MotorMSpeed_rads/1 -> Ku_EAngleSet_Caller/1

== system MDCC/DoCurCtr_sys/MDCC/FW ==
  FCN : TriggerPort  TriggerType=function-call  VariantControl=(inherit)  PortDimensions=1
  CDD_Gtm_UVW_SetFW : FunctionCaller  FunctionPrototype=PiIoHwSetInvState_C_SwsSet_DPO_UVW_FW()  InputArgumentSpecifications=<Enter example>  OutputArgumentSpecifications=<Enter example>

== system MDCC/DoCurCtr_sys/MDCC/IrmsCalc_Sys ==
  A_Element_Inlet : Inport
  B_Element_Inlet : Inport  Port=2
  C_Element_Inlet : Inport  Port=3
  Chart : Stateflow chart  TreatAsAtomicUnit=on
  Data Store Memory : DataStoreMemory  DataStoreName=Array_A  ReadBeforeWriteMsg=warning  WriteAfterWriteMsg=warning  WriteAfterReadMsg=warning  InitialValue=zeros(1000,1)  ShowAdditionalParam=off
  Data Store Memory1 : DataStoreMemory  DataStoreName=Array_B  ReadBeforeWriteMsg=warning  WriteAfterWriteMsg=warning  WriteAfterReadMsg=warning  InitialValue=zeros(1000,1)  ShowAdditionalParam=off
  Data Store Memory2 : DataStoreMemory  DataStoreName=Array_C  ReadBeforeWriteMsg=warning  WriteAfterWriteMsg=warning  WriteAfterReadMsg=warning  InitialValue=zeros(1000,1)  ShowAdditionalParam=off
  Data Store Read : DataStoreRead  DataStoreName=Array_A  IndexOptions=Index vector (dialog)  Indices=1  OutputSizes=1
  Data Store Read1 : DataStoreRead  DataStoreName=Array_B  IndexOptions=Index vector (dialog)  Indices=1  OutputSizes=1
  Data Store Read2 : DataStoreRead  DataStoreName=Array_C  IndexOptions=Index vector (dialog)  Indices=1  OutputSizes=1
  Enabled Subsystem : Subsystem  TreatAsAtomicUnit=on
  Gain : Gain  Gain=0.0001
  Gain1 : Gain  Gain=0.0001
  Gain2 : Gain  Gain=0.0001
  Product : Product
  Product1 : Product
  Product2 : Product
  Subsystem : Subsystem
  Subsystem1 : Subsystem
  Subsystem2 : Subsystem
  Subsystem3 : Subsystem
  A_Rms_Out : Outport
  B_Rms_Out : Outport  Port=2
  C_Rms_Out : Outport  Port=3
  wires:
  Subsystem/2(Vector) -> Subsystem2/1(Vector), Subsystem1/1(Vector)
  Subsystem1/1(Earliest_Element_A) -> Subsystem3/1(Earliest_Element_A)
  Subsystem3/1(A2_Rms) -> Enabled Subsystem/1(A2_Rms)
  Subsystem/1(RmsValueValid) -> Enabled Subsystem/Enable
  Product/1 -> Gain/1
  Subsystem1/2(Earliest_Element_B) -> Subsystem3/3(Earliest_Element_B)
  Subsystem1/3(Earliest_Element_C) -> Subsystem3/5(Earliest_Element_C)
  Product1/1 -> Gain1/1
  Product2/1 -> Gain2/1
  Subsystem3/2(B2_Rms) -> Enabled Subsystem/2(B2_Rms)
  Subsystem3/3(C2_Rms) -> Enabled Subsystem/3(C2_Rms)
  Enabled Subsystem/2(B_Rms_Out) -> B_Rms_Out/1
  Enabled Subsystem/1(A_Rms_Out) -> A_Rms_Out/1
  Enabled Subsystem/3(C_Rms_Out) -> C_Rms_Out/1
  Data Store Read/1 -> Subsystem1/2(PreArray_A)
  Data Store Read1/1 -> Subsystem1/3(PreArray_B)
  Data Store Read2/1 -> Subsystem1/4(PreArray_C)
  Chart/1(First()) -> [First]
  Chart/2(Second()) -> [Second]
  Chart/3(Thrid()) -> [Thrid]
  [First] -> Subsystem1/Trigger
  [Second] -> Subsystem2/Trigger
  [Thrid] -> Subsystem3/Trigger
  A_Element_Inlet/1 -> Product/2, Product/1
  B_Element_Inlet/1 -> Product1/2, Product1/1
  C_Element_Inlet/1 -> Product2/2, Product2/1
  Gain/1 -> Subsystem3/2(Element_Inlet_A), Subsystem2/2(Element_Inlet_A)
  Gain2/1 -> Subsystem3/6(Element_Inlet_C), Subsystem2/4(Element_Inlet_C)
  Gain1/1 -> Subsystem3/4(Element_Inlet_B), Subsystem2/3(Element_Inlet_B)

== system MDCC/DoCurCtr_sys/MDCC/MDCC_Debug_UaUb ==
  function : TriggerPort  TriggerType=function-call  VariantControl=Variant
  Constant : Constant  Value=KfMDCC_DebugUalphaVolCmd_V
  Constant1 : Constant  Value=KfMDCC_DebugUbetaVolCmd_V
  VfMDCC_UalphaVol_V : Outport
  VfMDCC_UbetaVol_V : Outport  Port=2
  wires:
  Constant/1 -> VfMDCC_UalphaVol_V/1
  Constant1/1 -> VfMDCC_UbetaVol_V/1

== system MDCC/DoCurCtr_sys/MDCC/MDCC_Debug_Us ==
  VuMDTM_PwmFrequency_Hz : Inport
  VfMDSP_MotorMSpeed_rads : Inport  Port=2
  function : TriggerPort  TriggerType=function-call  VariantControl=Variant
  EAngleOL1 : Subsystem
      settings: RTWSystemCode=Nonreusable function  RTWFcnNameOpts=Use subsystem name
  Product : Product
  Product1 : Product
  VolOL : Subsystem
  VfMDCC_UalphaVol_V : Outport
  VfMDCC_UbetaVol_V : Outport  Port=2
  wires:
  VuMDTM_PwmFrequency_Hz/1 -> EAngleOL1/1(VuMDTM_PwmFrequency_Hz)
  EAngleOL1/1(cos) -> Product/1
  VolOL/1(UsSlope) -> Product/2, Product1/2
  EAngleOL1/2(sin) -> Product1/1
  Product/1 -> VfMDCC_UalphaVol_V/1
  Product1/1 -> VfMDCC_UbetaVol_V/1
  VfMDSP_MotorMSpeed_rads/1 -> EAngleOL1/2(VfMDSP_MotorMSpeed_rads)

== system MDCC/DoCurCtr_sys/MDCC/PWMEn ==
  function : TriggerPort  VariantControl=(inherit)
  Constant1 : Constant  Value=true
  Function Caller : FunctionCaller  FunctionPrototype=PiIoHwSetInvState_C_Sws_UVW_PwmEnOutput(IoHwAbOpArg_PwmOutputEn)  InputArgumentSpecifications=boolean(0)
  wires:
  Constant1/1 -> Function Caller/1

== system MDCC/DoCurCtr_sys/MDCC/ResAngle_Sys ==
  VuMDSP_MotorPositionCnt_NULL_read : Inport  OutMin=[0]  OutMax=[4095]
  FCN : TriggerPort  TriggerType=function-call  VariantControl=(inherit)  PortDimensions=1
  Signal Copy : SignalConversion  OverrideOpt=off
  VuMDCC_MotorPositionCnt_NULL : Outport
  wires:
  Signal Copy/1 -> VuMDCC_MotorPositionCnt_NULL/1
  VuMDSP_MotorPositionCnt_NULL_read/1 -> Signal Copy/1

== system MDCC/DoCurCtr_sys/MDCC/SVM_Calc ==
  VfMDCC_UalphaVol_V : Inport
  VfMDCC_UbetaVol_V : Inport  Port=2
  VfMDCC_DCLinkVolUsed_V : Inport  Port=3
  VuMDTM_PwmFrequency_Hz : Inport  Port=4
  VfMDCC_dCur_A : Inport  Port=5
  VfMDCC_qCur_A : Inport  Port=6
  VfMDCM_IdRefVal_A : Inport  Port=7
  VfMDCM_IqRefVal_A : Inport  Port=8
  VuMDSP_MotorPositionCnt_NULL : Inport  Port=9  OutMin=[0]  OutMax=[4095]
  VfMDSP_MotorMSpeed_rads : Inport  Port=10
  uDcLink : Inport  Port=11
  function1 : TriggerPort  TriggerType=function-call  VariantControl=Variant
  Constant : Constant  Value=KbMDCC_DeadTimeCompEn_flg
  Data Type Conversion : DataTypeConversion  OutDataTypeStr=single
  DeadComp_Sys : Subsystem  TreatAsAtomicUnit=on
      settings: RTWSystemCode=Nonreusable function  RTWFcnNameOpts=Use subsystem name
  Delay : Delay  DelayLength=1
  MDSA : Subsystem  TreatAsAtomicUnit=on  RTWFcnName=MDSA  RTWFileName=MDSA
      settings: RTWSystemCode=Nonreusable function  RTWFcnNameOpts=User specified
  Switch : Switch  Criteria=u2 ~= 0
  Switch1 : Switch  Criteria=u2 ~= 0
  Switch2 : Switch  Criteria=u2 ~= 0
  VuMDTM_PwmFrequency_Hz1 : InportShadow  Port=4
  VfMDCC_PwmDutyCyclePhaseU_NULL : Outport
  VfMDCC_PwmDutyCyclePhaseV_NULL : Outport  Port=2
  VfMDCC_PwmDutyCyclePhaseW_NULL : Outport  Port=3
  VfMDCC_PWMDutyUDeadCompFINAL_NULL : Outport  Port=4
  VfMDCC_PWMDutyVDeadCompFINAL_NULL : Outport  Port=5
  VfMDCC_PWMDutyWDeadCompFINAL_NULL : Outport  Port=6
  wires:
  MDSA/1(VfMDSA_PwmDutyCyclePhaseU_NULL) -> Switch/3, VfMDCC_PwmDutyCyclePhaseU_NULL/1, DeadComp_Sys/1(U_Phase_Dyc)  "VfMDSA_PwmDutyCyclePhaseU_NULL"
  VfMDCC_UalphaVol_V/1 -> MDSA/1(VfMDCC_Ualpha_V)
  VuMDTM_PwmFrequency_Hz/1 -> MDSA/4(VuMDTM_PwmFrequency_Hz)
  MDSA/2(VfMDSA_PwmDutyCyclePhaseV_NULL) -> Switch1/3, VfMDCC_PwmDutyCyclePhaseV_NULL/1, DeadComp_Sys/2(V_Phase_Dyc)  "VfMDSA_PwmDutyCyclePhaseV_NULL"
  MDSA/3(VfMDSA_PwmDutyCyclePhaseW_NULL) -> Switch2/3, VfMDCC_PwmDutyCyclePhaseW_NULL/1, DeadComp_Sys/3(W_Phase_Dyc)  "VfMDSA_PwmDutyCyclePhaseW_NULL"
  VfMDCC_UbetaVol_V/1 -> MDSA/2(VfMDCC_Ubeta_V)
  VfMDCC_DCLinkVolUsed_V/1 -> MDSA/3(VfMDCC_DCLinkVolUsed_V)
  VfMDCC_dCur_A/1 -> DeadComp_Sys/6(IsdFb_A)
  VfMDCC_qCur_A/1 -> DeadComp_Sys/7(IsqFb_A)
  VfMDCM_IdRefVal_A/1 -> DeadComp_Sys/4(IsdDes_A)
  VfMDCM_IqRefVal_A/1 -> DeadComp_Sys/5(IsqDes_A)
  VuMDTM_PwmFrequency_Hz1/1 -> DeadComp_Sys/9(PwmFreq_Hz)
  Constant/1 -> Delay/1, DeadComp_Sys/Enable
  Switch/1 -> VfMDCC_PWMDutyUDeadCompFINAL_NULL/1
  Switch1/1 -> VfMDCC_PWMDutyVDeadCompFINAL_NULL/1
  Switch2/1 -> VfMDCC_PWMDutyWDeadCompFINAL_NULL/1
  VfMDSP_MotorMSpeed_rads/1 -> DeadComp_Sys/11(VfMDSP_MotorMSpeed_rads)
  uDcLink/1 -> DeadComp_Sys/10(uDcLink)
  Data Type Conversion/1 -> DeadComp_Sys/8(agPreRtrEl)
  VuMDSP_MotorPositionCnt_NULL/1 -> Data Type Conversion/1
  DeadComp_Sys/1(VfMDCC_PWMDutyUDeadCompFINAL_NULL) -> Switch/1  "VfMDCC_PWMDutyUDeadCompFINAL_NULL"
  DeadComp_Sys/2(VfMDCC_PWMDutyVDeadCompFINAL_NULL) -> Switch1/1  "VfMDCC_PWMDutyVDeadCompFINAL_NULL"
  DeadComp_Sys/3(VfMDCC_PWMDutyWDeadCompFINAL_NULL) -> Switch2/1  "VfMDCC_PWMDutyWDeadCompFINAL_NULL"
  Delay/1 -> Switch2/2, Switch1/2, Switch/2

== system MDCC/DoCurCtr_sys/MDCC/Simulink Function ==
  Ku_EAngleSet : TriggerPort  TriggerType=function-call  IsSimulinkFunction=on  FunctionName=Ku_EAngleSet  FunctionVisibility=scoped  VariantControl=(inherit)
  Data Type Conversion : DataTypeConversion  OutDataTypeStr=uint16  RndMeth=Zero
  Enabled Subsystem : Subsystem  TreatAsAtomicUnit=on
  Merge : Merge
  NOT : Logic  Operator=NOT  IconShape=distinctive  AllPortsSameDT=off  OutDataTypeStr=boolean
  Subsystem : Subsystem
  pi2_4096 : Gain  Gain=4096/2/pi  OutDataTypeStr=single
  Kf_SpdCmd_rads : ArgIn  DisableCoverage=on  OutDataTypeStr=single  ArgumentName=Kf_SpdCmd_rads
  Vu_PwmFrequency_Hz : ArgIn  DisableCoverage=on  Port=2  OutDataTypeStr=uint16  ArgumentName=Vu_PwmFrequency_Hz
  Ke_MotorPolePairsNum_NULL : ArgIn  DisableCoverage=on  Port=3  OutDataTypeStr=uint8  ArgumentName=Ke_MotorPolePairsNum_NULL
  Kb_SetEAngleFixValEn_flg : ArgIn  DisableCoverage=on  Port=4  OutDataTypeStr=boolean  ArgumentName=Kb_SetEAngleFixValEn_flg
  Kf_SetEAngle_Null : ArgIn  DisableCoverage=on  Port=5  OutMin=0  OutMax=360  OutDataTypeStr=single  ArgumentName=Kf_SetEAngle_Null
  Vu_AutoEAngle_NULL : ArgOut  DisableCoverage=on  OutDataTypeStr=uint16  ArgumentName=Vu_AutoEAngle_NULL
  wires:
  Ke_MotorPolePairsNum_NULL/1 -> Subsystem/1(Ke_MotorPolePairsNum_NULL)
  Kf_SpdCmd_rads/1 -> Subsystem/2(Kf_SpdCmd_rads)
  Vu_PwmFrequency_Hz/1 -> Subsystem/3(Vu_PwmFrequency_Hz)
  Subsystem/1(Vf_AutoEAngle_NULL) -> Merge/2
  Kb_SetEAngleFixValEn_flg/1 -> Enabled Subsystem/Enable, NOT/1
  NOT/1 -> Subsystem/Enable
  pi2_4096/1 -> Data Type Conversion/1
  Kf_SetEAngle_Null/1 -> Enabled Subsystem/1(Kf_SetEAngle_Null)
  Enabled Subsystem/1(Vf_AutoEAngle_NULL) -> Merge/1
  Merge/1 -> pi2_4096/1
  Data Type Conversion/1 -> Vu_AutoEAngle_NULL/1
